simulink model "WaterTankLevelControlDemo"  (R2026a)
settings: Solver=VariableStepAuto  StopTime=150
PreLoadFcn:
  | WaterTankLevelControlDemo_init
StopFcn:
  | watertank_stopfcn_export
values from neighbouring files (symbols this model uses):
  g_const = 9.81    [WaterTankLevelControlDemo_init.m]
  H0 = 0.3    [WaterTankLevelControlDemo_init.m]
  Kd_Level = 0    [WaterTankLevelControlDemo_init.m]    (also in export_batch_results.m = Kd_vals(kd_idx); watertank_export_from_out.m = Kd_vals(kd_idx); watertank_postsim_export.m = localGetVar(simIn, 'Kd_Level'); watertank_stopfcn_export.m = evalin('base', 'Kd_Level'))
  Ki_Level = 0.4    [WaterTankLevelControlDemo_init.m]    (also in export_batch_results.m = Ki_vals(ki_idx); watertank_export_from_out.m = Ki_vals(ki_idx); watertank_postsim_export.m = localGetVar(simIn, 'Ki_Level'); watertank_stopfcn_export.m = evalin('base', 'Ki_Level'))
  Kp_Level = 4    [WaterTankLevelControlDemo_init.m]    (also in export_batch_results.m = Kp_vals(kp_idx); watertank_export_from_out.m = Kp_vals(kp_idx); watertank_postsim_export.m = localGetVar(simIn, 'Kp_Level'); watertank_stopfcn_export.m = evalin('base', 'Kp_Level'))
  MaxValveArea = 5e-4    (= 0.0005)    [WaterTankLevelControlDemo_init.m]
  P_atm = 1e5    (= 100000)    [WaterTankLevelControlDemo_init.m]
  P_supply = 3e4    (= 30000)    [WaterTankLevelControlDemo_init.m]
  rho_water = 1000    [WaterTankLevelControlDemo_init.m]
libraries: fl_lib x7, nesl_utility x3, slpidlib x1
settings Model: Creator=yukky  LastModifiedBy=yukky

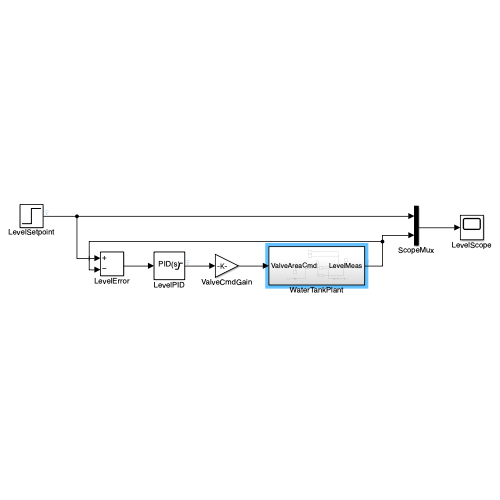
[thumbnail: Simulink's stored preview of the top-level diagram]
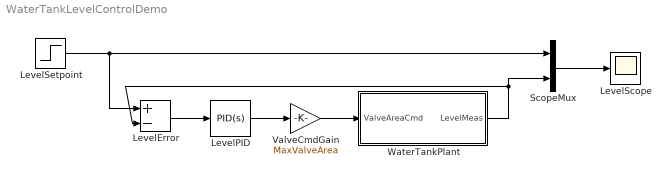
== system WaterTankLevelControlDemo ==
  LevelError : Sum  Inputs=+-
  LevelPID : slpidlib/PID Controller  Controller=PID  Form=Parallel  TimeDomain=Continuous-time  UseExternalTs=off  SampleTime=-1  IntegratorMethod=Forward Euler  FilterMethod=Forward Euler  ControllerParametersSource=internal  P=Kp_Level  I=Ki_Level  UseKiTs=off  D=Kd_Level  UseExternalDerivativeSource=off  N=100  UseFilter=on  TunerSelectOption=Transfer Function Based (PID Tuner App)  InitialConditionSource=internal  InitialConditionForIntegrator=0  InitialConditionForFilter=0  DifferentiatorICPrevScaledInput=0  ExternalReset=none  TrackingMode=off  Kt=1  LimitOutput=on  SatLimitsSource=internal  UpperSaturationLimit=1  LowerSaturationLimit=0  LinearizeAsGain=on  AntiWindupMode=back-calculation  Kb=1  LimitIntegrator=off  UpperIntegratorSaturationLimit=inf  LowerIntegratorSaturationLimit=-inf  POutMin=[]  POutMax=[]  IOutMin=[]  IOutMax=[]  DOutMin=[]  DOutMax=[]  NOutMin=[]  NOutMax=[]  SumOutMin=[]  SumOutMax=[]  SaturationOutMin=[]  SaturationOutMax=[]  PParamMin=[]  PParamMax=[]  IParamMin=[]  IParamMax=[]  DParamMin=[]  DParamMax=[]  NParamMin=[]  NParamMax=[]  KbParamMin=[]  KbParamMax=[]  KtParamMin=[]  KtParamMax=[]  KbOutMin=[]  KbOutMax=[]  KtOutMin=[]  KtOutMax=[]  IntegratorOutMin=[]  IntegratorOutMax=[]  FilterOutMin=[]  FilterOutMax=[]  SumI1OutMin=[]  SumI1OutMax=[]  SumI2OutMin=[]  SumI2OutMax=[]  SumI3OutMin=[]  SumI3OutMax=[]  SumI4OutMin=[]  SumI4OutMax=[]  SumDOutMin=[]  SumDOutMax=[]  DifferentiatorOutMin=[]  DifferentiatorOutMax=[]  FilterDiffOutCoefMin=[]  FilterDiffOutCoefMax=[]  ReciprocalOutMin=[]  ReciprocalOutMax=[]  SumDenOutMin=[]  SumDenOutMax=[]  SumNumOutMin=[]  SumNumOutMax=[]  DivideOutMin=[]  DivideOutMax=[]  UdiffTsProdOutMin=[]  UdiffTsProdOutMax=[]  NTsProdOutMin=[]  NTsProdOutMax=[]  UintegralTsProdOutMin=[]  UintegralTsProdOutMax=[]  UngainTsProdOutMin=[]  UngainTsProdOutMax=[]  ClampingZeroOutDataTypeStr=Inherit: Inherit via back propagation  ClampingZeroOutMin=[]  ClampingZeroOutMax=[]  FilterDenConstantOutDataTypeStr=Inherit: Inherit via back propagation  FilterDenConstantOutMin=[]  FilterDenConstantOutMax=[]  PCopyOutDataTypeStr=Inherit: Inherit via back propagation  PCopyOutMin=[]  PCopyOutMax=[]  NCopyOutDataTypeStr=Inherit: Inherit via back propagation  NCopyOutMin=[]  NCopyOutMax=[]  IntegratorContinuousStateAttributes=''  IntegratorStateMustResolveToSignalObject=off  IntegratorRTWStateStorageClass=Auto  FilterContinuousStateAttributes=''  FilterStateMustResolveToSignalObject=off  FilterRTWStateStorageClass=Auto  ParallelPVariant=InternalParameters  IdealPVariant=Disabled  IVariant=InternalParameters  DVariant=InternalParameters  IntegratorVariant=Continuous  SatVariant=Enabled  AWVariant=BackCalculation  PCopyVariant=Disabled  TRVariant=Disabled  FdbkBlocksVariant=Forward  IdealPFdbkVariant=Disabled  SatFdbkVariant=Disabled  DerivativeFilterVariant=ContFilter  NVariant=InternalParameters  NCopyVariant=Disabled  FilterICVariant=InternalICsFilter  IntegratorICVariant=InternalICs  ExternalResetVariant=Disabled  TRSumVariant=Passthrough  SumFdbkVariant=Disabled  SumVariant=Sum_PID  TsampFilterVariant=InternalTs  TsampNgainVariant=Passthrough  TsampIntegralVariant=Disabled_SignalSpec  ExternalSaturationOutDataTypeStr=Inherit: Same as second input  DerivativeSourceVariant=ErrorSignal  PreIntVariant=InternalPreInt
  LevelScope : Scope
      settings: ActiveDisplayYMinimum=0.1723109935597929  ActiveDisplayYMaximum=1.3901315907262959
  LevelSetpoint : Step  Time=20  InitialValue=H0  FinalValue=1.2  SampleTime=0
  ScopeMux : Mux  Inputs=2
  ValveCmdGain : Gain  Gain=MaxValveArea
  WaterTankPlant : Subsystem
  wires:
  LevelSetpoint/1 -> LevelError/1, ScopeMux/1
  WaterTankPlant/1(LevelMeas) -> LevelError/2, ScopeMux/2
  LevelError/1 -> LevelPID/1
  LevelPID/1 -> ValveCmdGain/1
  ValveCmdGain/1 -> WaterTankPlant/1(ValveAreaCmd)
  ScopeMux/1 -> LevelScope/1

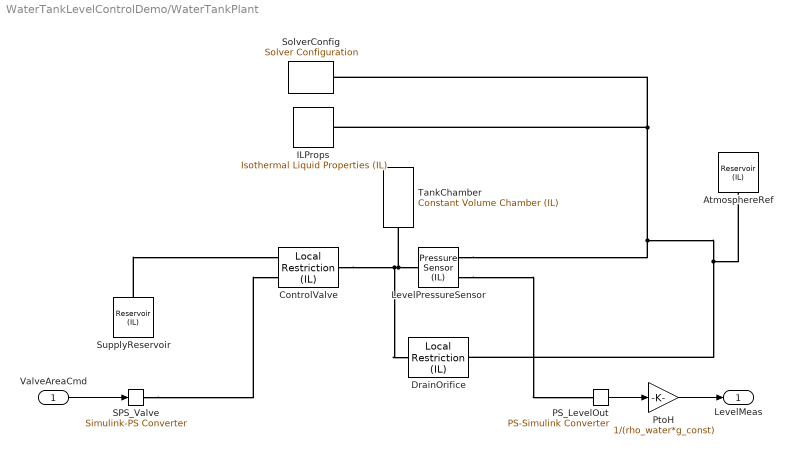
== system WaterTankLevelControlDemo/WaterTankPlant ==
  ValveAreaCmd : Inport
  AtmosphereRef : fl_lib/Isothermal Liquid/Elements/Reservoir (IL)  pressure_input=false  pressure_spec=foundation.enum.pressure_spec.specified  reservoir_pressure=P_atm Pa
  ControlValve : fl_lib/Isothermal Liquid/Elements/Local Restriction (IL)  restriction_type=foundation.enum.restriction_type.variable  restriction_area=1e-3 m^2  min_area=1e-8 m^2  max_area=MaxValveArea m^2  area=inf m^2  Cd=0.64  Re_c=150  pressure_recovery=false
  DrainOrifice : fl_lib/Isothermal Liquid/Elements/Local Restriction (IL)  restriction_type=foundation.enum.restriction_type.fixed  restriction_area=DrainArea m^2  min_area=1e-10 m^2  max_area=0.005 m^2  area=inf m^2  Cd=0.64  Re_c=150  pressure_recovery=false
  ILProps : fl_lib/Isothermal Liquid/Utilities/Isothermal Liquid Properties (IL)  rho_L_atm=998.21 kg/m^3  bulk_modulus_model=foundation.enum.bulk_modulus_model.const  beta_gain=6  beta_L_atm=beta_L Pa  nu_atm=1.0034e-6 m^2/s  p_atm=0.101325 MPa  p_min=1 Pa  properties_range_check=simscape.enum.assert.action.none  air_fraction=0.005  polytropic_index=1.0  rho_g_atm=1.225 kg/m^3  air_dissolution_model=false  p_crit=3 MPa
  LevelPressureSensor : fl_lib/Isothermal Liquid/Sensors/Pressure Sensor (IL)  pressure_measure=foundation.enum.pressure_measure.difference
  PS_LevelOut : nesl_utility/PS-Simulink Converter  PhysicalDomain=network_engine_domain  SubClassName=ps_output  LeftPortType=input  RightPortType=output  PseudoPeriodic=off  Frequencies=[]  VectorFormat=inherit  Unit=Pa  AffineConversion=off
  PtoH : Gain  Gain=1/(rho_water*g_const)
  SPS_Valve : nesl_utility/Simulink-PS Converter  PhysicalDomain=network_engine_domain  SubClassName=ps_input  LeftPortType=input  RightPortType=output  PseudoPeriodic=off  Frequencies=[]  NoiseDistribution=none  NoiseParameters=[]  Unit=m^2  AffineConversion=off  FilteringAndDerivatives=provide  SimscapeFilterOrder=1  InputFilterTimeConstant=0.001  UdotUserProvided=0
  SolverConfig : nesl_utility/Solver Configuration  PhysicalDomain=network_engine_domain  SubClassName=solver  LeftPortType=input  RightPortType=generic  Tones=[]  Harmonics=[]  SimulateNoise=off  Profile=off  UseLocalSampling=off  EnableSwitchedLinearOptims=on  FrequencyDomain=off  UseCCode=off  RelTol=0.001  AbsTol=0.001  MinStep=1e-09  ToWorkspace=off  RevertToSquareIcSolve=off  NumHomotopyIterations=100  PhasorMode=off  PhasorModeNumHarmonics=1  ConsistencySolver=NEWTON_XTOL_AFTER_FTOL  CanonicalOrdering=CANONICAL  OptimizeIntermediates=OPTIMIZED  IndexReductionMethod=DerivativeReplacement  DoDC=off  ResidualTolerance=1e-09  ConsistencyTolSource=GLOBAL  ConsistencyAbsTol=0.001  ConsistencyRelTol=0.001  ConsistencyTolFactor=0.001  UseLocalSolver=off  LocalSolverChoice=NE_BACKWARD_EULER_ADVANCER  ResolveIndetEquations=on  FunctionEvalNumThread=1  LocalSolverSampleTime=0.001  DoFixedCost=off  MaxNonlinIter=3  MaxModeIter=2  ComputeImpulses=off  ImpulseIterations=2  LinearAlgebra=auto  LinearAlgebraNumThread=0  EquationFormulation=NE_TIME_EF  DelaysMemoryBudget=1024  AutomaticFiltering=on  FilteringTimeConstant=0.001  PartitionStorageMethod=AS_NEEDED  PartitionMemoryBudget=1024  PartitionMethod=ROBUST  MultibodyUseLocalSolver=off  MultibodyLocalSolverChoice=ODE1  MultibodyLocalSolverSampleTime=0.001
  SupplyReservoir : fl_lib/Isothermal Liquid/Elements/Reservoir (IL)  pressure_input=false  pressure_spec=foundation.enum.pressure_spec.specified  reservoir_pressure=P_supply+P_atm Pa
  TankChamber : fl_lib/Isothermal Liquid/Elements/Constant Volume Chamber (IL)  volume=V_chamber m^3  p_I_specify=on  p_I_priority=High  p_I=P_atm+rho_water*g_const*H0 Pa  p_I_nominal_specify=off  p_I_nominal_value=1  p_I_nominal_unit=MPa
  LevelMeas : Outport
  wires:
  ValveAreaCmd/1 -> SPS_Valve/1
  PS_LevelOut/1 -> PtoH/1
  PtoH/1 -> LevelMeas/1
  connections:
  SPS_Valve/RConn1 -- ControlValve/LConn2
  LevelPressureSensor/RConn1 -- DrainOrifice/RConn1 -- AtmosphereRef/LConn1 -- SolverConfig/RConn1 -- ILProps/RConn1
  SupplyReservoir/LConn1 -- ControlValve/LConn1
  DrainOrifice/LConn1 -- LevelPressureSensor/LConn1 -- TankChamber/LConn1 -- ControlValve/RConn1
  LevelPressureSensor/RConn2 -- PS_LevelOut/LConn1
